simulink model "Model_3"  (R2022b)
settings: Solver=VariableStepAuto  StartTime=0.0  StopTime=10.0  RelTol=1e-3
libraries: arduinolib x3
settings Model: Creator=djand  LastModifiedBy=djand

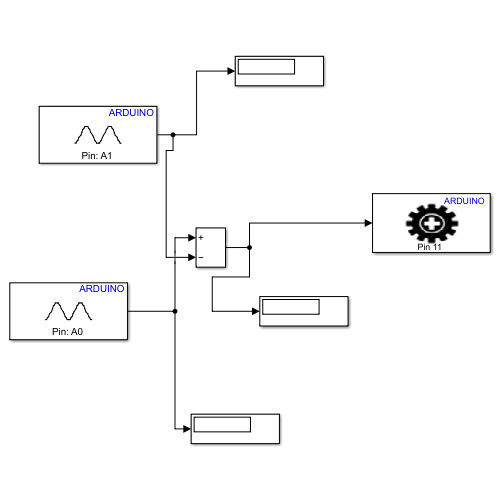
[thumbnail: Simulink's stored preview of the top-level diagram]
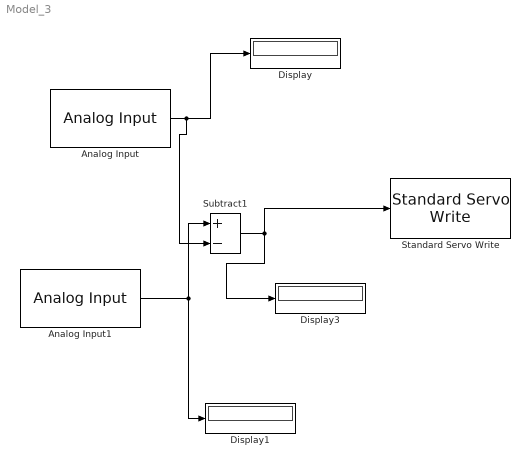
== system Model_3 ==
  Analog Input : arduinolib/Analog Input  pinNumber=1  ReadResultsOnly=off  ConversionTriggerSource=Software  ExternalTriggerType=uint32( 0 )  OutputDataType=uint16  EnableConversionCompleteNotify=off  EnableOuputStatus=off  SampleTime=0.1  blockPlatform=arduino
  Analog Input1 : arduinolib/Analog Input  pinNumber=0  ReadResultsOnly=off  ConversionTriggerSource=Software  ExternalTriggerType=uint32( 0 )  OutputDataType=uint16  EnableConversionCompleteNotify=off  EnableOuputStatus=off  SampleTime=0.1  blockPlatform=arduino
  Display : Display
  Display1 : Display
  Display3 : Display
      settings: Format=decimal (Stored Integer)
  Standard Servo Write : arduinolib/Standard Servo Write  pinNumber=11  ServoIndex=0  blockPlatform=arduino
  Subtract1 : Sum  Inputs=+-  SaturateOnIntegerOverflow=on  OutDataTypeStr=Inherit: Same as first input
  wires:
  Analog Input1/1 -> Display1/1, Subtract1/1
  Subtract1/1 -> Display3/1, Standard Servo Write/1
  Analog Input/1 -> Display/1, Subtract1/2
